simulink library "L_inf_allocation_lib"  (R2018b)
settings: Solver=VariableStepAuto  StartTime=0.0  StopTime=10.0  RelTol=1e-3
undefined symbols (not defined in the file): fswParams
settings Model: Creator=taylorreynolds  LastModifiedBy=Taylor

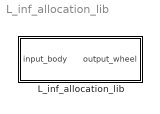
== system L_inf_allocation_lib ==
  L_inf_allocation_lib : Subsystem  TreatAsAtomicUnit=on
      settings: RTWFcnNameOpts=Use subsystem name  RTWFileNameOpts=Use subsystem name

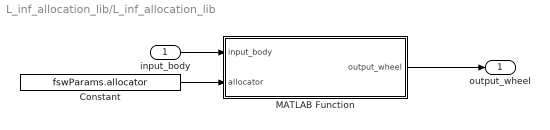
== system L_inf_allocation_lib/L_inf_allocation_lib ==
  input_body : Inport
  Constant : Constant  Value=fswParams.allocator  OutDataTypeStr=Bus: RWA
  MATLAB Function : MATLAB Function  TreatAsAtomicUnit=on
  output_wheel : Outport
  wires:
  input_body/1 -> MATLAB Function/1(input_body)
  MATLAB Function/1(output_wheel) -> output_wheel/1
  Constant/1 -> MATLAB Function/2(allocator)

== matlab function L_inf_allocation_lib/MATLAB Function ==
  data: input_body input double size=3; output_wheel output double size=4; allocator input Bus: RWA
function output_wheel = alloc_main(input_body,allocator)
%#codegen

val = 0.0;
id  = uint8(1);
w_facet = allocator.w_facet;
for k = 1:allocator.num_facet
   temp = abs( dot(w_facet(:,k),input_body) );
   if (temp > val)
       val = temp;
       id = k;
   end
end
facet = allocator.id_facet(id,:);
facet_complement = allocator.id_facet_complement(id,:);

w_hat_i = allocator.A_wheel2body(:,facet(1));
w_hat_j = allocator.A_wheel2body(:,facet(2));
w_ij    = w_facet(:,id);
g_ij    = allocator.g_facet(id);
inrm2   = allocator.inrm2(id);

H_0     = dot(w_ij,input_body);
w_i_H   = dot(w_hat_i,input_body);
w_j_H   = dot(w_hat_j,input_body);
w_i_j   = dot(w_hat_i,w_hat_j);

output_wheel = zeros(4,1);

output_wheel(facet(1)) = inrm2 * ( w_i_H - w_i_j*w_j_H ) - g_ij * H_0; 
output_wheel(facet(2)) = inrm2 * ( w_j_H - w_i_j*w_i_H ) - g_ij * H_0;
for k = facet_complement
    w_hat_k = allocator.A_wheel2body(:,k);
    output_wheel(k) = H_0 * sign( dot(w_hat_k,w_ij) );
end

end
